simulink model "rths_tp2b30ef9c_efc8_407a_bf56_5907fe18dc70"  (R2025b)
settings: Solver=ode4  StartTime=0.0  StopTime=40  FixedStep=dt  RelTol=1e-3
model workspace (MAT data in the model file):
  A1 = [0 0 0 0 0 0 0 0 0 0 0 0 ... (900 elements, 30x30)]
  A2 = [0  0  0  0  0  1  0  0  0  0; 0  0  0  0  0  0  1  0  0  0; 0  0  0  0  0  0  0  1  0  0; 0  0  0  0  0  0  0  0  1  0; 0  0  0  0  0  0  0  0  0  1; -6809.72287599  1725.02771323  -333.089032362  475.979287483  335.637011278  -10.3232478622  2.28107730426  -0.440457753921  0.629407598294  0.443827054501; 1725.02771323  -1275.41870211  -224.506613981  -485.535072622  -254.797165003  2.28107730426  -3.00500274123  -0.296874617074  -0.642043618248  -0.336929097325; -30247.7702549  -20387.4154373  -45657.3936355  -10111.0493928  -2173.61782727  -39.997909427  -26.9591440705  -61.6931704515  -13.3702694254  -2.87426703692; 43223.615115  -44091.374679  -10111.0493928  -48022.1598274  -10067.4687905  57.1564193959  -58.3038946694  -13.3702694254  -64.8202010776  -13.3126409467; 30479.1518777  -23138.096304  -2173.61782727  -10067.4687905  -25815.0707914  40.3038751599  -30.5964860379  -2.87426703692  -13.3126409467  -35.4548254345]
  A3 = [0 0 0 0 0 0 0 0 -6465.93985904 1514.25007638 -29949.4995057 42366.3776755 ... (256 elements, 16x16)]
  B1 = [0  0  0  0  0  0  0  0  0  0  0  0  0  0  0; 0  0  0  0  0  0  0  0  0  0  0  0  0  0  0; 0  0  0  0  0  0  0  0  0  0  0  0  0  0  0; 0  0  0  0  0  0  0  0  0  0  0  0  0  0  0; 0  0  0  0  0  0  0  0  0  0  0  0  0  0  0; 0  0  0  0  0  0  0  0  0  0  0  0  0  0  0; 0  0  0  0  0  0  0  0  0  0  0  0  0  0  0; 0  0  0  0  0  0  0  0  0  0  0  0  0  0  0; 0  0  0  0  0  0  0  0  0  0  0  0  0  0  0; 0  0  0  0  0  0  0  0  0  0  0  0  0  0  0; 0  0  0  0  0  0  0  0  0  0  0  0  0  0  0; 0  0  0  0  0  0  0  0  0  0  0  0  0  0  0; 0  0  0  0  0  0  0  0  0  0  0  0  0  0  0; 0  0  0  0  0  0  0  0  0  0  0  0  0  0  0; 0  0  0  0  0  0  0  0  0  0  0  0  0  0  0; 0.000162210458758  0  0  0  0  0  0  0  0  0  0  0  0  0  0; 0  0.0195741403137  0  0  0  0  0  0  0  0  0  0  0  0  0; 0  0  0.0147303099554  0  0  0  0  0  0  0  0  0  0  0  0; 0  0  0  0.0147303099554  0  0  0  0  0  0  0  0  0  0  0; 0  0  0  0  0.0195741403137  0  0  0  0  0  0  0  0  0  0; 0  0  0  0  0  0.000162210458758  0  0  0  0  0  0  0  0  0; 0  0  0  0  0  0  0.0195741403137  0  0  0  0  0  0  0  0; 0  0  0  0  0  0  0  0.0147303099554  0  0  0  0  0  0  0; 0  0  0  0  0  0  0  0  0.0147303099554  0  0  0  0  0  0; 0  0  0  0  0  0  0  0  0  0.0195741403137  0  0  0  0  0; 0  0  0  0  0  0  0  0  0  0  0.000162210458758  0  0  0  0; 0  0  0  0  0  0  0  0  0  0  0  0.0195741403137  0  0  0; 0  0  0  0  0  0  0  0  0  0  0  0  0.0147303099554  0  0; 0  0  0  0  0  0  0  0  0  0  0  0  0  0.0147303099554  0; 0  0  0  0  0  0  0  0  0  0  0  0  0  0  0.0195741403137]
  B2 = [0  0  0  0  0; 0  0  0  0  0; 0  0  0  0  0; 0  0  0  0  0; 0  0  0  0  0; 0.000162210458758  0  0  0  0; 0  0.000162210458758  0  0  0; 0  0  0.0147303099554  0  0; 0  0  0  0.0147303099554  0; 0  0  0  0  0.0147303099554]
  B3 = [0  0  0  0  0  0  0  0; 0  0  0  0  0  0  0  0; 0  0  0  0  0  0  0  0; 0  0  0  0  0  0  0  0; 0  0  0  0  0  0  0  0; 0  0  0  0  0  0  0  0; 0  0  0  0  0  0  0  0; 0  0  0  0  0  0  0  0; 0.000153222079678  -1.38864775191e-06  6.80539052363e-06  1.64914321893e-05  -2.57137705377e-05  0.00857679801195  -0.000293449983094  0.000726097409968; -1.38864775191e-06  0.000149515144127  1.93940221838e-05  -5.12172676809e-06  -3.82827328132e-05  0.00423910351833  -0.000212205388444  0.000534478402469; 6.80539052363e-06  1.93940221838e-05  0.0146353780333  5.09760170252e-06  8.11087485506e-05  -0.0644103990989  -0.000816445152791  5.37981551207e-05; 1.64914321893e-05  -5.12172676809e-06  5.09760170252e-06  0.0146828972607  1.89184773836e-05  0.00301816330771  0.0037908129159  -0.00354316274617; -2.57137705377e-05  -3.82827328132e-05  8.11087485506e-05  1.89184773836e-05  0.0145571946627  0.0536495512827  -0.00848725124143  0.00847023294881; 0.00857679801195  0.00423910351833  -0.0644103990989  0.00301816330771  0.0536495512827  2.11717274554  -0.0520147420295  0.0899270581681; -0.000293449983094  -0.000212205388444  -0.000816445152791  0.0037908129159  -0.00848725124143  -0.0520147420295  1.00698052503  -0.00826432567244; 0.000726097409968  0.000534478402469  5.37981551207e-05  -0.00354316274617  0.00847023294881  0.0899270581681  -0.00826432567244  1.01153242275]
  C1 = [1  0  0  0  0  0  0  0  0  0  0  0  0  0  0  0  0  0  0  0  0  0  0  0  0  0  0  0  0  0; 0  0  0  0  0  1  0  0  0  0  0  0  0  0  0  0  0  0  0  0  0  0  0  0  0  0  0  0  0  0; 0  0  0  0  0  0  0  0  0  0  1  0  0  0  0  0  0  0  0  0  0  0  0  0  0  0  0  0  0  0]
  C2 = [1  0  0  0  0  0  0  0  0  0; 0.719397421364  0.455029805905  -0.0548687646055  0.00094719287358  0.0504515218309  0  0  0  0  0; 0  1  0  0  0  0  0  0  0  0]
  C3 = [1  0  0  0  0  0  0  0  0  0  0  0  0  0  0  0; 0.719397421364  0.455029805905  -0.0548687646055  0.00094719287358  0.0504515218309  -0.0115996183931  0.000450409849156  -0.00105854789448  0  0  0  0  0  0  0  0; 0  1  0  0  0  0  0  0  0  0  0  0  0  0  0  0]
  D1 = [0  0  0  0  0  0  0  0  0  0  0  0  0  0  0; 0  0  0  0  0  0  0  0  0  0  0  0  0  0  0; 0  0  0  0  0  0  0  0  0  0  0  0  0  0  0]
  D2 = [0  0  0  0  0; 0  0  0  0  0; 0  0  0  0  0]
  D3 = [0  0  0  0  0  0  0  0; 0  0  0  0  0  0  0  0; 0  0  0  0  0  0  0  0]
  cb_force = [10599.793839; 8970.01227322; -338.256639094; 5.83928361236; 311.025085664; -71.5096824327; 2.7767004212; -6.52576845281]
  dt = 0.0009765625
  excitation_input = [0 0.0009765625 0.001953125 0.0029296875 0.00390625 0.0048828125 0.005859375 0.0068359375 0.0078125 0.0087890625 0.009765625 0.0107421875 ... (81922 elements, 40961x2)]
  full_force = [6164.83060128; 0; 0; 0; 0; 6164.83060128; 0; 0; 0; 0; 6164.83060128; 0; 0; 0; 0]
  guyan_force = [10599.793839; 8970.01227322; -338.256639094; 5.83928361236; 311.025085664]
settings Model: Creator=lenovo  LastModifiedBy=lenovo
settings DataIOCC: SaveOutput=off  SignalLogging=off  SaveTime=off

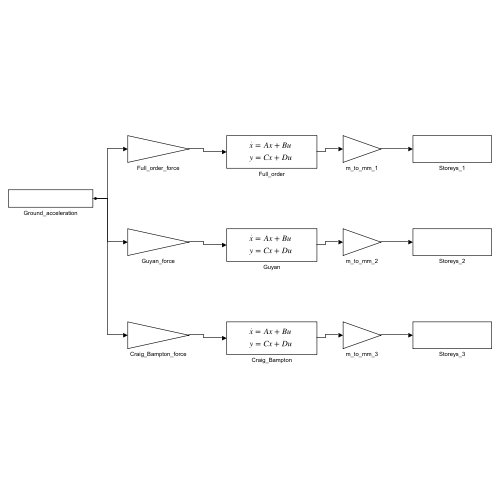
[thumbnail: Simulink's stored preview of the top-level diagram]
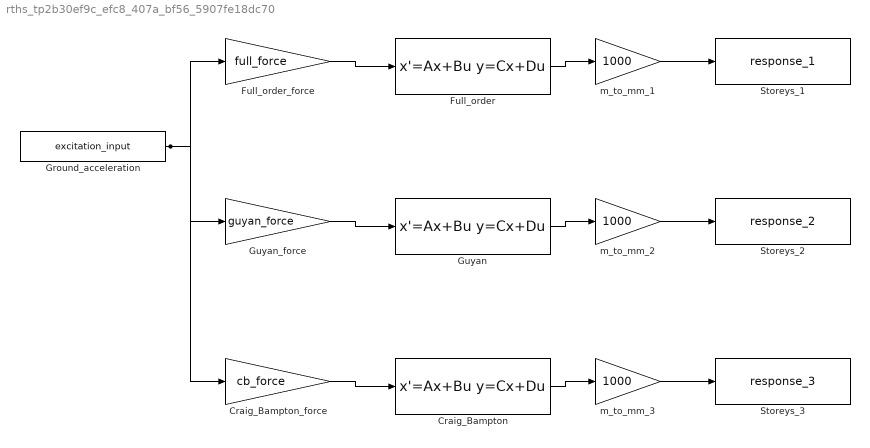
== system rths_tp2b30ef9c_efc8_407a_bf56_5907fe18dc70 ==
  Craig_Bampton : StateSpace  A=A3  B=B3  C=C3  D=D3  InitialCondition=0
  Craig_Bampton_force : Gain  Gain=cb_force
  Full_order : StateSpace  A=A1  B=B1  C=C1  D=D1  InitialCondition=0
  Full_order_force : Gain  Gain=full_force
  Ground_acceleration : FromWorkspace  VariableName=excitation_input  OutputAfterFinalValue=Holding final value
  Guyan : StateSpace  A=A2  B=B2  C=C2  D=D2  InitialCondition=0
  Guyan_force : Gain  Gain=guyan_force
  Storeys_1 : ToWorkspace  VariableName=response_1  SaveFormat=Timeseries  SampleTime=-1
  Storeys_2 : ToWorkspace  VariableName=response_2  SaveFormat=Timeseries  SampleTime=-1
  Storeys_3 : ToWorkspace  VariableName=response_3  SaveFormat=Timeseries  SampleTime=-1
  m_to_mm_1 : Gain  Gain=1000
  m_to_mm_2 : Gain  Gain=1000
  m_to_mm_3 : Gain  Gain=1000
  wires:
  Ground_acceleration/1 -> Full_order_force/1, Guyan_force/1, Craig_Bampton_force/1
  Full_order_force/1 -> Full_order/1
  Full_order/1 -> m_to_mm_1/1
  m_to_mm_1/1 -> Storeys_1/1
  Guyan_force/1 -> Guyan/1
  Guyan/1 -> m_to_mm_2/1
  m_to_mm_2/1 -> Storeys_2/1
  Craig_Bampton_force/1 -> Craig_Bampton/1
  Craig_Bampton/1 -> m_to_mm_3/1
  m_to_mm_3/1 -> Storeys_3/1
